simulink model "kamerol"  (R2021b)
settings: Solver=VariableStepAuto  StartTime=0.0  StopTime=10.0  RelTol=1e-3
undefined symbols (not defined in the file): admireDB
libraries: simulink_extras x104, simulink x24, sharedutil x1
(part 10 of 14)

== system kamerol/Aerodynamics/PitchMomentCoefficient/MachRegion2/Cpmdle/Subsystem ==
  angleOfAttack_deg : Inport
  dE : Inport  Port=2
  dN : Inport  Port=3
  tflow : Inport  Port=4
  tfhigh : Inport  Port=5
  lef_deg : Inport  Port=6
  " mach_nd_cnst" : Constant  Value=0.5
  CPMDLAL_ALFA : Lookup_n-D  NumberOfTableDimensions=1  BreakpointsForDimension1=admireDB.aerodata_sym.CPMDLAL.breakpoints.ALFA  BreakpointsForDimension3=[5, 7]  Table=admireDB.aerodata_sym.CPMDLAL.newTable  ExtrapMethod=Clip  InternalRulePriority=Speed  RndMeth=Simplest  InputSameDT=on
  CPMDLDEA_DE_ALFA : Lookup_n-D  BreakpointsForDimension1=admireDB.aerodata_sym.CPMDLDEA.breakpoints.ALFA  BreakpointsForDimension2=admireDB.aerodata_sym.CPMDLDEA.breakpoints.DE  BreakpointsForDimension3=[5, 7]  Table=admireDB.aerodata_sym.CPMDLDEA.newTable  ExtrapMethod=Clip  InternalRulePriority=Speed  RndMeth=Simplest  InputSameDT=on
      settings: InputPortMap=u0,u1
  CPMDLDNA_DN_ALFA : Lookup_n-D  BreakpointsForDimension1=admireDB.aerodata_sym.CPMDLDNA.breakpoints.ALFA  BreakpointsForDimension2=admireDB.aerodata_sym.CPMDLDNA.breakpoints.DN  BreakpointsForDimension3=[5, 7]  Table=admireDB.aerodata_sym.CPMDLDNA.newTable  ExtrapMethod=Clip  InternalRulePriority=Speed  RndMeth=Simplest  InputSameDT=on
      settings: InputPortMap=u0,u1
  CPMMDLEA_ALFA_DLE_M : Lookup_n-D  NumberOfTableDimensions=3  BreakpointsForDimension1=admireDB.aerodata_sym.CPMMDLEA.breakpoints.ALFA  BreakpointsForDimension2=admireDB.aerodata_sym.CPMMDLEA.breakpoints.DLE  BreakpointsForDimension3=admireDB.aerodata_sym.CPMMDLEA.breakpoints.M  Table=admireDB.aerodata_sym.CPMMDLEA.newTable  ExtrapMethod=Clip  InternalRulePriority=Speed  RndMeth=Simplest  InputSameDT=on
      settings: InputPortMap=u0,u1,u2
  Constant : Constant  Value=1/27
  Product : Product  Inputs=4
  Product1 : Product
  Sum : Sum  Inputs=+++
  Sum1 : Sum  Inputs=|++
  Out1 : Outport
  wires:
  Product1/1 -> Sum1/2
  Sum1/1 -> Out1/1
  tfhigh/1 -> Product1/1
  CPMMDLEA_ALFA_DLE_M/1 -> Product1/2
  angleOfAttack_deg/1 -> CPMDLAL_ALFA/1, CPMDLDEA_DE_ALFA/1, CPMDLDNA_DN_ALFA/1, CPMMDLEA_ALFA_DLE_M/1
  lef_deg/1 -> Product/3, CPMMDLEA_ALFA_DLE_M/2
  " mach_nd_cnst"/1 -> CPMMDLEA_ALFA_DLE_M/3
  tflow/1 -> Product/1
  dE/1 -> CPMDLDEA_DE_ALFA/2
  CPMDLDNA_DN_ALFA/1 -> Sum/3
  Sum/1 -> Product/2
  CPMDLAL_ALFA/1 -> Sum/1
  CPMDLDEA_DE_ALFA/1 -> Sum/2
  Product/1 -> Sum1/1
  dN/1 -> CPMDLDNA_DN_ALFA/2
  Constant/1 -> Product/4

== system kamerol/Aerodynamics/PitchMomentCoefficient/MachRegion2/Cpmdle/Subsystem1 ==
  qacorr : Inport
  mach_nd : Inport  Port=2
  CPMEDLEI_QA_M : Lookup_n-D  BreakpointsForDimension1=admireDB.aerodata_sym.CPMEDLEI.breakpoints.M  BreakpointsForDimension2=admireDB.aerodata_sym.CPMEDLEI.breakpoints.QA  BreakpointsForDimension3=[5, 7]  Table=admireDB.aerodata_sym.CPMEDLEI.newTable  ExtrapMethod=Clip  InternalRulePriority=Speed  RndMeth=Simplest  InputSameDT=on
      settings: InputPortMap=u0,u1
  CPMEDLEY_QA_M : Lookup_n-D  BreakpointsForDimension1=admireDB.aerodata_sym.CPMEDLEY.breakpoints.M  BreakpointsForDimension2=admireDB.aerodata_sym.CPMEDLEY.breakpoints.QA  BreakpointsForDimension3=[5, 7]  Table=admireDB.aerodata_sym.CPMEDLEY.newTable  ExtrapMethod=Clip  InternalRulePriority=Speed  RndMeth=Simplest  InputSameDT=on
      settings: InputPortMap=u0,u1
  Sum1 : Sum  Inputs=|++
  Out1 : Outport
  wires:
  mach_nd/1 -> CPMEDLEY_QA_M/1, CPMEDLEI_QA_M/1
  CPMEDLEY_QA_M/1 -> Sum1/2
  CPMEDLEI_QA_M/1 -> Sum1/1
  qacorr/1 -> CPMEDLEY_QA_M/2, CPMEDLEI_QA_M/2
  Sum1/1 -> Out1/1

== system kamerol/Aerodynamics/PitchMomentCoefficient/MachRegion2/Cpmdn/CPMDNAL_CPMMDNA ==
  dN : Inport
  angleOfAttack_deg : Inport  Port=2
  tflow : Inport  Port=3
  tfhigh : Inport  Port=4
  CPMDNAL_DN_ALFA : Lookup_n-D  BreakpointsForDimension1=admireDB.aerodata_sym.CPMDNAL.breakpoints.ALFA  BreakpointsForDimension2=admireDB.aerodata_sym.CPMDNAL.breakpoints.DN  BreakpointsForDimension3=[5, 7]  Table=admireDB.aerodata_sym.CPMDNAL.newTable  ExtrapMethod=Clip  InternalRulePriority=Speed  RndMeth=Simplest  InputSameDT=on
      settings: InputPortMap=u0,u1
  CPMMDNA_ALFA_DN_M : Lookup_n-D  NumberOfTableDimensions=3  BreakpointsForDimension1=admireDB.aerodata_sym.CPMMDNA.breakpoints.ALFA  BreakpointsForDimension2=admireDB.aerodata_sym.CPMMDNA.breakpoints.DN  BreakpointsForDimension3=admireDB.aerodata_sym.CPMMDNA.breakpoints.M  Table=admireDB.aerodata_sym.CPMMDNA.newTable  ExtrapMethod=Clip  InternalRulePriority=Speed  RndMeth=Simplest  InputSameDT=on
      settings: InputPortMap=u0,u1,u2
  Product : Product
  Product1 : Product
  Sum : Sum  Inputs=|++
  mach_nd_cnst : Constant  Value=0.5
  Out1 : Outport
  wires:
  Product1/1 -> Sum/2
  tfhigh/1 -> Product1/1
  Product/1 -> Sum/1
  tflow/1 -> Product/2
  mach_nd_cnst/1 -> CPMMDNA_ALFA_DN_M/3
  Sum/1 -> Out1/1
  angleOfAttack_deg/1 -> CPMDNAL_DN_ALFA/1, CPMMDNA_ALFA_DN_M/1
  CPMDNAL_DN_ALFA/1 -> Product/1
  dN/1 -> CPMDNAL_DN_ALFA/2, CPMMDNA_ALFA_DN_M/2
  CPMMDNA_ALFA_DN_M/1 -> Product1/2

== system kamerol/Aerodynamics/PitchMomentCoefficient/MachRegion2/Cpmq/Subsystem ==
  tflow : Inport
  angleOfAttack_deg : Inport  Port=2
  dN : Inport  Port=3
  tfhigh : Inport  Port=4
  CPMQAL_ALFA : Lookup_n-D  NumberOfTableDimensions=1  BreakpointsForDimension1=admireDB.aerodata_sym.CPMQAL.breakpoints.ALFA  BreakpointsForDimension3=[5, 7]  Table=admireDB.aerodata_sym.CPMQAL.newTable  ExtrapMethod=Clip  InternalRulePriority=Speed  RndMeth=Simplest  InputSameDT=on
  CPMQAM_ALFA_M : Lookup_n-D  BreakpointsForDimension1=admireDB.aerodata_sym.CPMQAM.breakpoints.M  BreakpointsForDimension2=admireDB.aerodata_sym.CPMQAM.breakpoints.ALFA  BreakpointsForDimension3=[5, 7]  Table=admireDB.aerodata_sym.CPMQAM.newTable  ExtrapMethod=Clip  InternalRulePriority=Speed  RndMeth=Simplest  InputSameDT=on
      settings: InputPortMap=u0,u1
  CPMQDNAL_DN_ALFA : Lookup_n-D  BreakpointsForDimension1=admireDB.aerodata_sym.CPMQDNAL.breakpoints.ALFA  BreakpointsForDimension2=admireDB.aerodata_sym.CPMQDNAL.breakpoints.DN  BreakpointsForDimension3=[5, 7]  Table=admireDB.aerodata_sym.CPMQDNAL.newTable  ExtrapMethod=Clip  InternalRulePriority=Speed  RndMeth=Simplest  InputSameDT=on
      settings: InputPortMap=u0,u1
  Product1 : Product
  Product2 : Product
  Sum : Sum  Inputs=++|
  Sum1 : Sum  Inputs=|++
  mach_nd_cnst : Constant  Value=0.5
  Out1 : Outport
  wires:
  dN/1 -> CPMQDNAL_DN_ALFA/2
  tfhigh/1 -> Product2/2
  Sum1/1 -> Out1/1
  tflow/1 -> Product1/1
  angleOfAttack_deg/1 -> CPMQAM_ALFA_M/2, CPMQDNAL_DN_ALFA/1, CPMQAL_ALFA/1
  Product2/1 -> Sum1/2
  CPMQAM_ALFA_M/1 -> Product2/1
  CPMQAL_ALFA/1 -> Sum/1
  mach_nd_cnst/1 -> CPMQAM_ALFA_M/1
  Sum/1 -> Product1/2
  Product1/1 -> Sum1/1
  CPMQDNAL_DN_ALFA/1 -> Sum/2

== system kamerol/Aerodynamics/PitchMomentCoefficient/MachRegion3/Cpmdei/Subsystem ==
  dEI : Inport
  angleOfAttack_deg : Inport  Port=2
  eieff : Inport  Port=3
  mach_nd : Inport  Port=4
  CPMMDEA_ALFA_DE_M : Lookup_n-D  NumberOfTableDimensions=3  BreakpointsForDimension1=admireDB.aerodata_sym.CPMMDEA.breakpoints.ALFA  BreakpointsForDimension2=admireDB.aerodata_sym.CPMMDEA.breakpoints.DE  BreakpointsForDimension3=admireDB.aerodata_sym.CPMMDEA.breakpoints.M  Table=admireDB.aerodata_sym.CPMMDEA.newTable  ExtrapMethod=Clip  InternalRulePriority=Speed  RndMeth=Simplest  InputSameDT=on
      settings: InputPortMap=u0,u1,u2
  CPMMDEA_ALFA_DE_M1 : Lookup_n-D  NumberOfTableDimensions=3  BreakpointsForDimension1=admireDB.aerodata_sym.CPMMDEA.breakpoints.ALFA  BreakpointsForDimension2=admireDB.aerodata_sym.CPMMDEA.breakpoints.DE  BreakpointsForDimension3=admireDB.aerodata_sym.CPMMDEA.breakpoints.M  Table=admireDB.aerodata_sym.CPMMDEA.newTable  ExtrapMethod=Clip  InternalRulePriority=Speed  RndMeth=Simplest  InputSameDT=on
      settings: InputPortMap=u0,u1,u2
  Constant : Constant  Value=0
  Product : Product
  Sum : Sum  Inputs=|+-
  Out1 : Outport
  wires:
  Constant/1 -> CPMMDEA_ALFA_DE_M1/2
  mach_nd/1 -> CPMMDEA_ALFA_DE_M1/3, CPMMDEA_ALFA_DE_M/3
  eieff/1 -> Product/2
  angleOfAttack_deg/1 -> CPMMDEA_ALFA_DE_M/1, CPMMDEA_ALFA_DE_M1/1
  Sum/1 -> Product/1
  CPMMDEA_ALFA_DE_M1/1 -> Sum/2
  CPMMDEA_ALFA_DE_M/1 -> Sum/1
  Product/1 -> Out1/1
  dEI/1 -> CPMMDEA_ALFA_DE_M/2

== system kamerol/Aerodynamics/PitchMomentCoefficient/MachRegion3/Cpmdey/Subsystem ==
  dEY : Inport
  angleOfAttack_deg : Inport  Port=2
  eoeff : Inport  Port=3
  mach_nd : Inport  Port=4
  CPMMDEA_ALFA_DE_M : Lookup_n-D  NumberOfTableDimensions=3  BreakpointsForDimension1=admireDB.aerodata_sym.CPMMDEA.breakpoints.ALFA  BreakpointsForDimension2=admireDB.aerodata_sym.CPMMDEA.breakpoints.DE  BreakpointsForDimension3=admireDB.aerodata_sym.CPMMDEA.breakpoints.M  Table=admireDB.aerodata_sym.CPMMDEA.newTable  ExtrapMethod=Clip  InternalRulePriority=Speed  RndMeth=Simplest  InputSameDT=on
      settings: InputPortMap=u0,u1,u2
  CPMMDEA_ALFA_DE_M1 : Lookup_n-D  NumberOfTableDimensions=3  BreakpointsForDimension1=admireDB.aerodata_sym.CPMMDEA.breakpoints.ALFA  BreakpointsForDimension2=admireDB.aerodata_sym.CPMMDEA.breakpoints.DE  BreakpointsForDimension3=admireDB.aerodata_sym.CPMMDEA.breakpoints.M  Table=admireDB.aerodata_sym.CPMMDEA.newTable  ExtrapMethod=Clip  InternalRulePriority=Speed  RndMeth=Simplest  InputSameDT=on
      settings: InputPortMap=u0,u1,u2
  Constant : Constant  Value=0
  Product : Product
  Sum : Sum  Inputs=|+-
  Out1 : Outport
  wires:
  dEY/1 -> CPMMDEA_ALFA_DE_M/2
  Product/1 -> Out1/1
  CPMMDEA_ALFA_DE_M/1 -> Sum/1
  CPMMDEA_ALFA_DE_M1/1 -> Sum/2
  Sum/1 -> Product/1
  angleOfAttack_deg/1 -> CPMMDEA_ALFA_DE_M1/1, CPMMDEA_ALFA_DE_M/1
  eoeff/1 -> Product/2
  mach_nd/1 -> CPMMDEA_ALFA_DE_M/3, CPMMDEA_ALFA_DE_M1/3
  Constant/1 -> CPMMDEA_ALFA_DE_M1/2

== system kamerol/Aerodynamics/PitchMomentCoefficient/MachRegion3/Cpmdle/Subsystem1 ==
  <qacorr> : Inport
  <mach_nd> : Inport  Port=2
  CPMEDLEI_QA_M : Lookup_n-D  BreakpointsForDimension1=admireDB.aerodata_sym.CPMEDLEI.breakpoints.M  BreakpointsForDimension2=admireDB.aerodata_sym.CPMEDLEI.breakpoints.QA  BreakpointsForDimension3=[5, 7]  Table=admireDB.aerodata_sym.CPMEDLEI.newTable  ExtrapMethod=Clip  InternalRulePriority=Speed  RndMeth=Simplest  InputSameDT=on
      settings: InputPortMap=u0,u1
  CPMEDLEY_QA_M : Lookup_n-D  BreakpointsForDimension1=admireDB.aerodata_sym.CPMEDLEY.breakpoints.M  BreakpointsForDimension2=admireDB.aerodata_sym.CPMEDLEY.breakpoints.QA  BreakpointsForDimension3=[5, 7]  Table=admireDB.aerodata_sym.CPMEDLEY.newTable  ExtrapMethod=Clip  InternalRulePriority=Speed  RndMeth=Simplest  InputSameDT=on
      settings: InputPortMap=u0,u1
  Sum1 : Sum  Inputs=|++
  Out1 : Outport
  wires:
  <mach_nd>/1 -> CPMEDLEY_QA_M/1, CPMEDLEI_QA_M/1
  CPMEDLEY_QA_M/1 -> Sum1/2
  CPMEDLEI_QA_M/1 -> Sum1/1
  <qacorr>/1 -> CPMEDLEY_QA_M/2, CPMEDLEI_QA_M/2
  Sum1/1 -> Out1/1

== system kamerol/Aerodynamics/RollMomentCoefficient/MachRegion1/Crmbasic/Crmbasic_ ==
  angleOfAttack_deg : Inport
  Abs : Abs
  CRMZERO_ALFA : Lookup_n-D  NumberOfTableDimensions=1  BreakpointsForDimension1=admireDB.aerodata_asym_ext.CRMZERO.breakpoints.ALFA  BreakpointsForDimension3=[5, 7]  Table=admireDB.aerodata_asym_ext.CRMZERO.newTable  ExtrapMethod=Clip  InternalRulePriority=Speed  RndMeth=Simplest  InputSameDT=on
  Crmbasic : Outport
  wires:
  Abs/1 -> CRMZERO_ALFA/1
  angleOfAttack_deg/1 -> Abs/1
  CRMZERO_ALFA/1 -> Crmbasic/1

== system kamerol/Aerodynamics/RollMomentCoefficient/MachRegion1/Crmbde/Crmbde_ ==
  angleOfAttack_deg : Inport
  dN : Inport  Port=2
  dEI : Inport  Port=3
  angleOfSideslip_deg : Inport  Port=4
  dEY : Inport  Port=5
  eieff : Inport  Port=6
  eoeff : Inport  Port=7
  Abs : Abs
  CRMDEB_ALFA_DN_DE_BETA : Lookup_n-D  NumberOfTableDimensions=4  BreakpointsForDimension1=admireDB.aerodata_asym_ext.CRMDEB.breakpoints.ALFA  BreakpointsForDimension2=admireDB.aerodata_asym_ext.CRMDEB.breakpoints.DN  BreakpointsForDimension3=admireDB.aerodata_asym_ext.CRMDEB.breakpoints.DE  BreakpointsForDimension4=admireDB.aerodata_asym_ext.CRMDEB.breakpoints.BETA  Table=admireDB.aerodata_asym_ext.CRMDEB.newTable  ExtrapMethod=Clip  InternalRulePriority=Speed  RndMeth=Simplest  InputSameDT=on
      settings: InputPortMap=u0,u1,u2,u3
  CRMDEB_ALFA_DN_DE_BETA_1 : Lookup_n-D  NumberOfTableDimensions=4  BreakpointsForDimension1=admireDB.aerodata_asym_ext.CRMDEB.breakpoints.ALFA  BreakpointsForDimension2=admireDB.aerodata_asym_ext.CRMDEB.breakpoints.DN  BreakpointsForDimension3=admireDB.aerodata_asym_ext.CRMDEB.breakpoints.DE  BreakpointsForDimension4=admireDB.aerodata_asym_ext.CRMDEB.breakpoints.BETA  Table=admireDB.aerodata_asym_ext.CRMDEB.newTable  ExtrapMethod=Clip  InternalRulePriority=Speed  RndMeth=Simplest  InputSameDT=on
      settings: InputPortMap=u0,u1,u2,u3
  Product : Product  Inputs=**
  Product1 : Product  Inputs=**
  Product2 : Product
  Sign : Signum
  Sum : Sum  Inputs=|++
  Crmbde : Outport
  wires:
  dEY/1 -> CRMDEB_ALFA_DN_DE_BETA_1/3
  dEI/1 -> CRMDEB_ALFA_DN_DE_BETA/3
  dN/1 -> CRMDEB_ALFA_DN_DE_BETA_1/2, CRMDEB_ALFA_DN_DE_BETA/2
  angleOfAttack_deg/1 -> CRMDEB_ALFA_DN_DE_BETA_1/1, CRMDEB_ALFA_DN_DE_BETA/1
  Sign/1 -> Product2/1
  Product2/1 -> Crmbde/1
  Product1/1 -> Sum/2
  Product/1 -> Sum/1
  Sum/1 -> Product2/2
  eoeff/1 -> Product1/1
  eieff/1 -> Product/2
  CRMDEB_ALFA_DN_DE_BETA_1/1 -> Product1/2
  CRMDEB_ALFA_DN_DE_BETA/1 -> Product/1
  Abs/1 -> CRMDEB_ALFA_DN_DE_BETA_1/4, CRMDEB_ALFA_DN_DE_BETA/4
  angleOfSideslip_deg/1 -> Abs/1, Sign/1

== system kamerol/Aerodynamics/RollMomentCoefficient/MachRegion1/Crmbdle/Crmbdle_ ==
  dLE : Inport
  angleOfSideslip_deg : Inport  Port=2
  dEI : Inport  Port=3
  angleOfAttack_deg : Inport  Port=4
  dEY : Inport  Port=5
  eieff : Inport  Port=6
  eoeff : Inport  Port=7
  Abs : Abs
  CRMDLEB_ALFA_DE_BETA_DLE : Lookup_n-D  NumberOfTableDimensions=4  BreakpointsForDimension1=admireDB.aerodata_asym_ext.CRMDLEB.breakpoints.ALFA  BreakpointsForDimension2=admireDB.aerodata_asym_ext.CRMDLEB.breakpoints.DE  BreakpointsForDimension3=admireDB.aerodata_asym_ext.CRMDLEB.breakpoints.BETA  BreakpointsForDimension4=admireDB.aerodata_asym_ext.CRMDLEB.breakpoints.DLE  Table=admireDB.aerodata_asym_ext.CRMDLEB.newTable  ExtrapMethod=Clip  InternalRulePriority=Speed  RndMeth=Simplest  InputSameDT=on
      settings: InputPortMap=u0,u1,u2,u3
  CRMDLEB_ALFA_DE_BETA_DLE_1 : Lookup_n-D  NumberOfTableDimensions=4  BreakpointsForDimension1=admireDB.aerodata_asym_ext.CRMDLEB.breakpoints.ALFA  BreakpointsForDimension2=admireDB.aerodata_asym_ext.CRMDLEB.breakpoints.DE  BreakpointsForDimension3=admireDB.aerodata_asym_ext.CRMDLEB.breakpoints.BETA  BreakpointsForDimension4=admireDB.aerodata_asym_ext.CRMDLEB.breakpoints.DLE  Table=admireDB.aerodata_asym_ext.CRMDLEB.newTable  ExtrapMethod=Clip  InternalRulePriority=Speed  RndMeth=Simplest  InputSameDT=on
      settings: InputPortMap=u0,u1,u2,u3
  Product1 : Product  Inputs=**
  Product2 : Product  Inputs=**
  Product3 : Product
  Sign : Signum
  Sum : Sum  Inputs=|++
  Crmbdle : Outport
  wires:
  dEY/1 -> CRMDLEB_ALFA_DE_BETA_DLE_1/2
  dEI/1 -> CRMDLEB_ALFA_DE_BETA_DLE/2
  Abs/1 -> CRMDLEB_ALFA_DE_BETA_DLE_1/3, CRMDLEB_ALFA_DE_BETA_DLE/3
  dLE/1 -> CRMDLEB_ALFA_DE_BETA_DLE_1/4, CRMDLEB_ALFA_DE_BETA_DLE/4
  CRMDLEB_ALFA_DE_BETA_DLE/1 -> Product1/1
  eoeff/1 -> Product2/1
  Product1/1 -> Sum/1
  Sum/1 -> Product3/2
  CRMDLEB_ALFA_DE_BETA_DLE_1/1 -> Product2/2
  Sign/1 -> Product3/1
  eieff/1 -> Product1/2
  Product2/1 -> Sum/2
  angleOfSideslip_deg/1 -> Abs/1, Sign/1
  angleOfAttack_deg/1 -> CRMDLEB_ALFA_DE_BETA_DLE_1/1, CRMDLEB_ALFA_DE_BETA_DLE/1
  Product3/1 -> Crmbdle/1

== system kamerol/Aerodynamics/RollMomentCoefficient/MachRegion1/Crmbdn/Crmbdn_ ==
  angleOfAttack_deg : Inport
  dN : Inport  Port=2
  angleOfSideslip_deg : Inport  Port=3
  Abs : Abs
  CRMDNB_ALFA_DN_BETA : Lookup_n-D  NumberOfTableDimensions=3  BreakpointsForDimension1=admireDB.aerodata_asym_ext.CRMDNB.breakpoints.ALFA  BreakpointsForDimension2=admireDB.aerodata_asym_ext.CRMDNB.breakpoints.DN  BreakpointsForDimension3=admireDB.aerodata_asym_ext.CRMDNB.breakpoints.BETA  Table=admireDB.aerodata_asym_ext.CRMDNB.newTable  ExtrapMethod=Clip  InternalRulePriority=Speed  RndMeth=Simplest  InputSameDT=on
      settings: InputPortMap=u0,u1,u2
  Product : Product
  Sign : Signum
  Crmbdn : Outport
  wires:
  Sign/1 -> Product/2
  CRMDNB_ALFA_DN_BETA/1 -> Product/1
  angleOfSideslip_deg/1 -> Abs/1, Sign/1
  angleOfAttack_deg/1 -> CRMDNB_ALFA_DN_BETA/1
  dN/1 -> CRMDNB_ALFA_DN_BETA/2
  Abs/1 -> CRMDNB_ALFA_DN_BETA/3
  Product/1 -> Crmbdn/1

== system kamerol/Aerodynamics/RollMomentCoefficient/MachRegion1/Crmbeta/Crmbeta_ ==
  angleOfSideslip_deg : Inport
  angleOfAttack_deg : Inport  Port=2
  qacorr : Inport  Port=3
  mach_nd : Inport  Port=4
  Abs : Abs
  CRMBAL_BETA_ALFA : Lookup_n-D  BreakpointsForDimension1=admireDB.aerodata_asym_ext.CRMBAL.breakpoints.ALFA  BreakpointsForDimension2=admireDB.aerodata_asym_ext.CRMBAL.breakpoints.BETA  BreakpointsForDimension3=[5, 7]  Table=admireDB.aerodata_asym_ext.CRMBAL.newTable  ExtrapMethod=Clip  InternalRulePriority=Speed  RndMeth=Simplest  InputSameDT=on
      settings: InputPortMap=u0,u1
  CRMEB_QA_M : Lookup_n-D  BreakpointsForDimension1=admireDB.aerodata_asym_ext.CRMEB.breakpoints.M  BreakpointsForDimension2=admireDB.aerodata_asym_ext.CRMEB.breakpoints.QA  BreakpointsForDimension3=[5, 7]  Table=admireDB.aerodata_asym_ext.CRMEB.newTable  ExtrapMethod=Clip  InternalRulePriority=Speed  RndMeth=Simplest  InputSameDT=on
      settings: InputPortMap=u0,u1
  Degrees to Radians : simulink_extras/Transformations/Degrees to Radians
  Product : Product
  Product1 : Product
  Sign : Signum
  Sum : Sum  Inputs=|++
  Crmbeta : Outport
  wires:
  Sum/1 -> Crmbeta/1
  Product1/1 -> Sum/2
  Degrees to Radians/1 -> Product1/1
  CRMEB_QA_M/1 -> Product1/2
  Product/1 -> Sum/1
  Abs/1 -> CRMBAL_BETA_ALFA/2
  Sign/1 -> Product/1
  CRMBAL_BETA_ALFA/1 -> Product/2
  angleOfSideslip_deg/1 -> Abs/1, Sign/1, Degrees to Radians/1
  mach_nd/1 -> CRMEB_QA_M/1
  angleOfAttack_deg/1 -> CRMBAL_BETA_ALFA/1
  qacorr/1 -> CRMEB_QA_M/2

== system kamerol/Aerodynamics/RollMomentCoefficient/MachRegion1/Crmbetad/Crmbetad_ ==
  angleOfAttack_deg : Inport
  betad : Inport  Port=2
  CRMBDL_ALFA : Lookup_n-D  NumberOfTableDimensions=1  BreakpointsForDimension1=admireDB.aerodata_asym_ext.CRMBDL.breakpoints.ALFA  BreakpointsForDimension3=[5, 7]  Table=admireDB.aerodata_asym_ext.CRMBDL.newTable  ExtrapMethod=Clip  InternalRulePriority=Speed  RndMeth=Simplest  InputSameDT=on
  Product : Product  Inputs=**
  Crmbetad : Outport
  wires:
  angleOfAttack_deg/1 -> CRMBDL_ALFA/1
  Product/1 -> Crmbetad/1
  CRMBDL_ALFA/1 -> Product/1
  betad/1 -> Product/2

== system kamerol/Aerodynamics/RollMomentCoefficient/MachRegion1/Crmblg/Crmblg_ ==
  dLG : Inport
  angleOfAttack_deg : Inport  Port=2
  angleOfSideslip_deg : Inport  Port=3
  CRMBLST_NG_DOOR_ALFA : Lookup_n-D  BreakpointsForDimension1=admireDB.aerodata_asym_ext.CRMBLST.breakpoints.ALFA  BreakpointsForDimension2=admireDB.aerodata_asym_ext.CRMBLST.breakpoints.NG_DOOR  BreakpointsForDimension3=[5, 7]  Table=admireDB.aerodata_asym_ext.CRMBLST.newTable  ExtrapMethod=Clip  InternalRulePriority=Speed  RndMeth=Simplest  InputSameDT=on
      settings: InputPortMap=u0,u1
  Degrees to Radians : simulink_extras/Transformations/Degrees to Radians
  Product : Product  Inputs=3
  Crmblg : Outport
  wires:
  Degrees to Radians/1 -> Product/3
  CRMBLST_NG_DOOR_ALFA/1 -> Product/2
  dLG/1 -> CRMBLST_NG_DOOR_ALFA/2, Product/1
  angleOfAttack_deg/1 -> CRMBLST_NG_DOOR_ALFA/1
  Product/1 -> Crmblg/1
  angleOfSideslip_deg/1 -> Degrees to Radians/1

== system kamerol/Aerodynamics/RollMomentCoefficient/MachRegion1/Crmdai/Crmdai_ ==
  dAI : Inport
  angleOfAttack_deg : Inport  Port=2
  dEI : Inport  Port=3
  eieff : Inport  Port=4
  qacorr : Inport  Port=5
  mach_nd : Inport  Port=6
  Abs : Abs
  CRMDAAL_DA_ALFA : Lookup_n-D  BreakpointsForDimension1=admireDB.aerodata_asym_ext.CRMDAAL.breakpoints.ALFA  BreakpointsForDimension2=admireDB.aerodata_asym_ext.CRMDAAL.breakpoints.DA  BreakpointsForDimension3=[5, 7]  Table=admireDB.aerodata_asym_ext.CRMDAAL.newTable  ExtrapMethod=Clip  InternalRulePriority=Speed  RndMeth=Simplest  InputSameDT=on
      settings: InputPortMap=u0,u1
  CRMDAL_DE_ALFA : Lookup_n-D  BreakpointsForDimension1=admireDB.aerodata_asym_ext.CRMDAL.breakpoints.ALFA  BreakpointsForDimension2=admireDB.aerodata_asym_ext.CRMDAL.breakpoints.DE  BreakpointsForDimension3=[5, 7]  Table=admireDB.aerodata_asym_ext.CRMDAL.newTable  ExtrapMethod=Clip  InternalRulePriority=Speed  RndMeth=Simplest  InputSameDT=on
      settings: InputPortMap=u0,u1
  CRMDAL_DE_ALFA_1 : Lookup_n-D  BreakpointsForDimension1=admireDB.aerodata_asym_ext.CRMDAL.breakpoints.ALFA  BreakpointsForDimension2=admireDB.aerodata_asym_ext.CRMDAL.breakpoints.DE  BreakpointsForDimension3=[5, 7]  Table=admireDB.aerodata_asym_ext.CRMDAL.newTable  ExtrapMethod=Clip  InternalRulePriority=Speed  RndMeth=Simplest  InputSameDT=on
      settings: InputPortMap=u0,u1
  CRMEDAI_QA_M : Lookup_n-D  BreakpointsForDimension1=admireDB.aerodata_asym_ext.CRMEDAI.breakpoints.M  BreakpointsForDimension2=admireDB.aerodata_asym_ext.CRMEDAI.breakpoints.QA  BreakpointsForDimension3=[5, 7]  Table=admireDB.aerodata_asym_ext.CRMEDAI.newTable  ExtrapMethod=Clip  InternalRulePriority=Speed  RndMeth=Simplest  InputSameDT=on
      settings: InputPortMap=u0,u1
  Degrees to Radians : simulink_extras/Transformations/Degrees to Radians
  Product : Product
  Product1 : Product
  Product2 : Product  Inputs=3
  Sign : Signum
  Sum : Sum  Inputs=|+-
  Sum1 : Sum  Inputs=|++
  dE_cnst : Constant  Value=0.0
  Crmdai : Outport
  wires:
  CRMEDAI_QA_M/1 -> Product2/3
  qacorr/1 -> CRMEDAI_QA_M/2
  mach_nd/1 -> CRMEDAI_QA_M/1
  eieff/1 -> Product2/2
  Sum1/1 -> Product2/1
  Product/1 -> Sum1/2
  Product1/1 -> Sum1/1
  Sign/1 -> Product1/1
  CRMDAAL_DA_ALFA/1 -> Product1/2
  Degrees to Radians/1 -> Product/1
  Sum/1 -> Product/2
  CRMDAL_DE_ALFA_1/1 -> Sum/2
  CRMDAL_DE_ALFA/1 -> Sum/1
  dEI/1 -> CRMDAL_DE_ALFA/2
  dE_cnst/1 -> CRMDAL_DE_ALFA_1/2
  dAI/1 -> Abs/1, Sign/1, Degrees to Radians/1
  Abs/1 -> CRMDAAL_DA_ALFA/2
  angleOfAttack_deg/1 -> CRMDAAL_DA_ALFA/1, CRMDAL_DE_ALFA_1/1, CRMDAL_DE_ALFA/1
  Product2/1 -> Crmdai/1

== system kamerol/Aerodynamics/RollMomentCoefficient/MachRegion1/Crmdaib/Crmdaib_ ==
  angleOfAttack_deg : Inport
  dAI : Inport  Port=2
  angleOfSideslip_deg : Inport  Port=3
  eieff : Inport  Port=4
  Abs : Abs
  Abs1 : Abs
  Abs2 : Abs
  CRMDABAL_ALFA : Lookup_n-D  NumberOfTableDimensions=1  BreakpointsForDimension1=admireDB.aerodata_asym_ext.CRMDABAL.breakpoints.ALFA  BreakpointsForDimension3=[5, 7]  Table=admireDB.aerodata_asym_ext.CRMDABAL.newTable  ExtrapMethod=Clip  InternalRulePriority=Speed  RndMeth=Simplest  InputSameDT=on
  Constant : Constant  Value=30
  Constant1 : Constant  Value=20
  Product : Product  Inputs=**/*/*
  Crmdaib : Outport
  wires:
  eieff/1 -> Product/6
  Abs2/1 -> Product/4
  Constant1/1 -> Product/5
  angleOfSideslip_deg/1 -> Abs2/1
  Constant/1 -> Product/3
  Abs1/1 -> Product/2
  Abs/1 -> CRMDABAL_ALFA/1
  dAI/1 -> Abs1/1
  CRMDABAL_ALFA/1 -> Product/1
  angleOfAttack_deg/1 -> Abs/1
  Product/1 -> Crmdaib/1

== system kamerol/Aerodynamics/RollMomentCoefficient/MachRegion1/Crmday/Crmday_ ==
  dAY : Inport
  angleOfAttack_deg : Inport  Port=2
  dEY : Inport  Port=3
  eoeff : Inport  Port=4
  qacorr : Inport  Port=5
  mach_nd : Inport  Port=6
  Abs : Abs
  CRMDAAL_DA_ALFA : Lookup_n-D  BreakpointsForDimension1=admireDB.aerodata_asym_ext.CRMDAAL.breakpoints.ALFA  BreakpointsForDimension2=admireDB.aerodata_asym_ext.CRMDAAL.breakpoints.DA  BreakpointsForDimension3=[5, 7]  Table=admireDB.aerodata_asym_ext.CRMDAAL.newTable  ExtrapMethod=Clip  InternalRulePriority=Speed  RndMeth=Simplest  InputSameDT=on
      settings: InputPortMap=u0,u1
  CRMDAL_DE_ALFA : Lookup_n-D  BreakpointsForDimension1=admireDB.aerodata_asym_ext.CRMDAL.breakpoints.ALFA  BreakpointsForDimension2=admireDB.aerodata_asym_ext.CRMDAL.breakpoints.DE  BreakpointsForDimension3=[5, 7]  Table=admireDB.aerodata_asym_ext.CRMDAL.newTable  ExtrapMethod=Clip  InternalRulePriority=Speed  RndMeth=Simplest  InputSameDT=on
      settings: InputPortMap=u0,u1
  CRMDAL_DE_ALFA_1 : Lookup_n-D  BreakpointsForDimension1=admireDB.aerodata_asym_ext.CRMDAL.breakpoints.ALFA  BreakpointsForDimension2=admireDB.aerodata_asym_ext.CRMDAL.breakpoints.DE  BreakpointsForDimension3=[5, 7]  Table=admireDB.aerodata_asym_ext.CRMDAL.newTable  ExtrapMethod=Clip  InternalRulePriority=Speed  RndMeth=Simplest  InputSameDT=on
      settings: InputPortMap=u0,u1
  CRMEDAY_QA_M : Lookup_n-D  BreakpointsForDimension1=admireDB.aerodata_asym_ext.CRMEDAY.breakpoints.M  BreakpointsForDimension2=admireDB.aerodata_asym_ext.CRMEDAY.breakpoints.QA  BreakpointsForDimension3=[5, 7]  Table=admireDB.aerodata_asym_ext.CRMEDAY.newTable  ExtrapMethod=Clip  InternalRulePriority=Speed  RndMeth=Simplest  InputSameDT=on
      settings: InputPortMap=u0,u1
  Degrees to Radians : simulink_extras/Transformations/Degrees to Radians
  Product : Product
  Product1 : Product
  Product2 : Product  Inputs=3
  Sign : Signum
  Sum : Sum  Inputs=|+-
  Sum1 : Sum  Inputs=|++
  dE_cnst : Constant  Value=0.0
  Crmdai : Outport
  wires:
  dE_cnst/1 -> CRMDAL_DE_ALFA_1/2
  Product2/1 -> Crmdai/1
  angleOfAttack_deg/1 -> CRMDAL_DE_ALFA_1/1, CRMDAL_DE_ALFA/1, CRMDAAL_DA_ALFA/1
  Abs/1 -> CRMDAAL_DA_ALFA/2
  dAY/1 -> Abs/1, Sign/1, Degrees to Radians/1
  dEY/1 -> CRMDAL_DE_ALFA/2
  CRMDAL_DE_ALFA/1 -> Sum/1
  CRMDAL_DE_ALFA_1/1 -> Sum/2
  Sum/1 -> Product/2
  Degrees to Radians/1 -> Product/1
  CRMDAAL_DA_ALFA/1 -> Product1/2
  Sign/1 -> Product1/1
  Product1/1 -> Sum1/1
  Product/1 -> Sum1/2
  Sum1/1 -> Product2/1
  eoeff/1 -> Product2/2
  qacorr/1 -> CRMEDAY_QA_M/2
  mach_nd/1 -> CRMEDAY_QA_M/1
  CRMEDAY_QA_M/1 -> Product2/3

== system kamerol/Aerodynamics/RollMomentCoefficient/MachRegion1/Crmdayb/Crmdaib_ ==
  angleOfAttack_deg : Inport
  dAY : Inport  Port=2
  angleOfSideslip_deg : Inport  Port=3
  eoeff : Inport  Port=4
  Abs : Abs
  Abs1 : Abs
  Abs2 : Abs
  CRMDABAL_ALFA : Lookup_n-D  NumberOfTableDimensions=1  BreakpointsForDimension1=admireDB.aerodata_asym_ext.CRMDABAL.breakpoints.ALFA  BreakpointsForDimension3=[5, 7]  Table=admireDB.aerodata_asym_ext.CRMDABAL.newTable  ExtrapMethod=Clip  InternalRulePriority=Speed  RndMeth=Simplest  InputSameDT=on
  Constant : Constant  Value=30
  Constant1 : Constant  Value=20
  Product : Product  Inputs=**/*/*
  Crmdaib : Outport
  wires:
  Product/1 -> Crmdaib/1
  angleOfAttack_deg/1 -> Abs/1
  CRMDABAL_ALFA/1 -> Product/1
  dAY/1 -> Abs1/1
  Abs/1 -> CRMDABAL_ALFA/1
  Abs1/1 -> Product/2
  Constant/1 -> Product/3
  angleOfSideslip_deg/1 -> Abs2/1
  Constant1/1 -> Product/5
  Abs2/1 -> Product/4
  eoeff/1 -> Product/6

== system kamerol/Aerodynamics/RollMomentCoefficient/MachRegion1/Crmdna/Crmdna_ ==
  dNE : Inport
  angleOfAttack_deg : Inport  Port=2
  dNA : Inport  Port=3
  CRMDNAAL_DNE_ALFA : Lookup_n-D  BreakpointsForDimension1=admireDB.aerodata_asym_ext.CRMDNAAL.breakpoints.ALFA  BreakpointsForDimension2=admireDB.aerodata_asym_ext.CRMDNAAL.breakpoints.DNE  BreakpointsForDimension3=[5, 7]  Table=admireDB.aerodata_asym_ext.CRMDNAAL.newTable  ExtrapMethod=Clip  InternalRulePriority=Speed  RndMeth=Simplest  InputSameDT=on
      settings: InputPortMap=u0,u1
  Degrees to Radians : simulink_extras/Transformations/Degrees to Radians
  Product : Product  Inputs=**
  Crmdna : Outport
  wires:
  Degrees to Radians/1 -> Product/2
  CRMDNAAL_DNE_ALFA/1 -> Product/1
  dNA/1 -> Degrees to Radians/1
  angleOfAttack_deg/1 -> CRMDNAAL_DNE_ALFA/1
  dNE/1 -> CRMDNAAL_DNE_ALFA/2
  Product/1 -> Crmdna/1

== system kamerol/Aerodynamics/RollMomentCoefficient/MachRegion1/Crmdr/Crmdr_ ==
  angleOfAttack_deg : Inport
  dR : Inport  Port=2
  angleOfSideslip_deg : Inport  Port=3
  qacorr : Inport  Port=4
  mach_nd : Inport  Port=5
  Abs : Abs
  CRMBDRAL_ALFA_DR_BETA : Lookup_n-D  NumberOfTableDimensions=3  BreakpointsForDimension1=admireDB.aerodata_asym_ext.CRMBDRAL.breakpoints.ALFA  BreakpointsForDimension2=admireDB.aerodata_asym_ext.CRMBDRAL.breakpoints.DR  BreakpointsForDimension3=admireDB.aerodata_asym_ext.CRMBDRAL.breakpoints.BETA  Table=admireDB.aerodata_asym_ext.CRMBDRAL.newTable  ExtrapMethod=Clip  InternalRulePriority=Speed  RndMeth=Simplest  InputSameDT=on
      settings: InputPortMap=u0,u1,u2
  CRMEDR_QA_M : Lookup_n-D  BreakpointsForDimension1=admireDB.aerodata_asym_ext.CRMEDR.breakpoints.M  BreakpointsForDimension2=admireDB.aerodata_asym_ext.CRMEDR.breakpoints.QA  BreakpointsForDimension3=[5, 7]  Table=admireDB.aerodata_asym_ext.CRMEDR.newTable  ExtrapMethod=Clip  InternalRulePriority=Speed  RndMeth=Simplest  InputSameDT=on
      settings: InputPortMap=u0,u1
  Product : Product
  Crmdr : Outport
  wires:
  CRMBDRAL_ALFA_DR_BETA/1 -> Product/1
  CRMEDR_QA_M/1 -> Product/2
  angleOfAttack_deg/1 -> CRMBDRAL_ALFA_DR_BETA/1
  angleOfSideslip_deg/1 -> Abs/1
  dR/1 -> CRMBDRAL_ALFA_DR_BETA/2
  Abs/1 -> CRMBDRAL_ALFA_DR_BETA/3
  qacorr/1 -> CRMEDR_QA_M/2
  mach_nd/1 -> CRMEDR_QA_M/1
  Product/1 -> Crmdr/1

== system kamerol/Aerodynamics/RollMomentCoefficient/MachRegion1/Crmp/Crmp_ ==
  dN : Inport
  angleOfAttack_deg : Inport  Port=2
  qacorr : Inport  Port=3
  mach_nd : Inport  Port=4
  pc : Inport  Port=5
  CRMEP_QA_M : Lookup_n-D  BreakpointsForDimension1=admireDB.aerodata_asym_ext.CRMEP.breakpoints.M  BreakpointsForDimension2=admireDB.aerodata_asym_ext.CRMEP.breakpoints.QA  BreakpointsForDimension3=[5, 7]  Table=admireDB.aerodata_asym_ext.CRMEP.newTable  ExtrapMethod=Clip  InternalRulePriority=Speed  RndMeth=Simplest  InputSameDT=on
      settings: InputPortMap=u0,u1
  CRMPAL_DN_ALFA : Lookup_n-D  BreakpointsForDimension1=admireDB.aerodata_asym_ext.CRMPAL.breakpoints.ALFA  BreakpointsForDimension2=admireDB.aerodata_asym_ext.CRMPAL.breakpoints.DN  BreakpointsForDimension3=[5, 7]  Table=admireDB.aerodata_asym_ext.CRMPAL.newTable  ExtrapMethod=Clip  InternalRulePriority=Speed  RndMeth=Simplest  InputSameDT=on
      settings: InputPortMap=u0,u1
  Product : Product  Inputs=3
  Crmp : Outport
  wires:
  Product/1 -> Crmp/1
  pc/1 -> Product/2
  CRMEP_QA_M/1 -> Product/3
  CRMPAL_DN_ALFA/1 -> Product/1
  angleOfAttack_deg/1 -> CRMPAL_DN_ALFA/1
  dN/1 -> CRMPAL_DN_ALFA/2
  mach_nd/1 -> CRMEP_QA_M/1
  qacorr/1 -> CRMEP_QA_M/2

== system kamerol/Aerodynamics/RollMomentCoefficient/MachRegion1/Crmpbeta/Crmpbeta_ ==
  angleOfSideslip_deg : Inport
  angleOfAttack_deg : Inport  Port=2
  pc : Inport  Port=3
  Abs : Abs
  CRMPBA_BETA_ALFA : Lookup_n-D  BreakpointsForDimension1=admireDB.aerodata_asym_ext.CRMPBA.breakpoints.ALFA  BreakpointsForDimension2=admireDB.aerodata_asym_ext.CRMPBA.breakpoints.BETA  BreakpointsForDimension3=[5, 7]  Table=admireDB.aerodata_asym_ext.CRMPBA.newTable  ExtrapMethod=Clip  InternalRulePriority=Speed  RndMeth=Simplest  InputSameDT=on
      settings: InputPortMap=u0,u1
  Product : Product  Inputs=**
  Crmpbeta : Outport
  wires:
  Abs/1 -> CRMPBA_BETA_ALFA/2
  CRMPBA_BETA_ALFA/1 -> Product/1
  angleOfSideslip_deg/1 -> Abs/1
  angleOfAttack_deg/1 -> CRMPBA_BETA_ALFA/1
  pc/1 -> Product/2
  Product/1 -> Crmpbeta/1

== system kamerol/Aerodynamics/RollMomentCoefficient/MachRegion1/Crmr/Crmr_ ==
  dN : Inport
  angleOfAttack_deg : Inport  Port=2
  rc : Inport  Port=3
  CRMRAL_DN_ALFA : Lookup_n-D  BreakpointsForDimension1=admireDB.aerodata_asym_ext.CRMRAL.breakpoints.ALFA  BreakpointsForDimension2=admireDB.aerodata_asym_ext.CRMRAL.breakpoints.DN  BreakpointsForDimension3=[5, 7]  Table=admireDB.aerodata_asym_ext.CRMRAL.newTable  ExtrapMethod=Clip  InternalRulePriority=Speed  RndMeth=Simplest  InputSameDT=on
      settings: InputPortMap=u0,u1
  Product : Product  Inputs=**
  Crmr : Outport
  wires:
  CRMRAL_DN_ALFA/1 -> Product/1
  angleOfAttack_deg/1 -> CRMRAL_DN_ALFA/1
  dN/1 -> CRMRAL_DN_ALFA/2
  Product/1 -> Crmr/1
  rc/1 -> Product/2

== system kamerol/Aerodynamics/RollMomentCoefficient/MachRegion1/Crmrbeta/Crmrbeta_ ==
  angleOfSideslip_deg : Inport
  angleOfAttack_deg : Inport  Port=2
  rc : Inport  Port=3
  Abs : Abs
  CRMRBA_BETA_ALFA : Lookup_n-D  BreakpointsForDimension1=admireDB.aerodata_asym_ext.CRMRBA.breakpoints.ALFA  BreakpointsForDimension2=admireDB.aerodata_asym_ext.CRMRBA.breakpoints.BETA  BreakpointsForDimension3=[5, 7]  Table=admireDB.aerodata_asym_ext.CRMRBA.newTable  ExtrapMethod=Clip  InternalRulePriority=Speed  RndMeth=Simplest  InputSameDT=on
      settings: InputPortMap=u0,u1
  Product : Product  Inputs=**
  Crmrbeta : Outport
  wires:
  Abs/1 -> CRMRBA_BETA_ALFA/2
  angleOfSideslip_deg/1 -> Abs/1
  angleOfAttack_deg/1 -> CRMRBA_BETA_ALFA/1
  rc/1 -> Product/2
  Product/1 -> Crmrbeta/1
  CRMRBA_BETA_ALFA/1 -> Product/1

== system kamerol/Aerodynamics/RollMomentCoefficient/MachRegion1/Crmrde/Crmrde_ ==
  mach_nd : Inport
  angleOfAttack_deg : Inport  Port=2
  rc : Inport  Port=3
  dEI : Inport  Port=4
  eieff : Inport  Port=5
  dey : Inport  Port=6
  eoeff : Inport  Port=7
  CRMRDEM_M : Lookup_n-D  NumberOfTableDimensions=1  BreakpointsForDimension1=admireDB.aerodata_asym_ext.CRMRDEM.breakpoints.M  BreakpointsForDimension3=[5, 7]  Table=admireDB.aerodata_asym_ext.CRMRDEM.newTable  ExtrapMethod=Clip  InternalRulePriority=Speed  RndMeth=Simplest  InputSameDT=on
  CRMRKA_ALFA : Lookup_n-D  NumberOfTableDimensions=1  BreakpointsForDimension1=admireDB.aerodata_asym_ext.CRMRKA.breakpoints.ALFA  BreakpointsForDimension3=[5, 7]  Table=admireDB.aerodata_asym_ext.CRMRKA.newTable  ExtrapMethod=Clip  InternalRulePriority=Speed  RndMeth=Simplest  InputSameDT=on
  Constant : Constant  Value=1/30
  Constant1 : Constant  Value=1/30
  Product : Product  Inputs=****
  Product1 : Product  Inputs=3
  Product2 : Product  Inputs=3
  Sum : Sum  Inputs=|++
  Crmrbeta : Outport
  wires:
  Sum/1 -> Product/4
  Product2/1 -> Sum/2
  Product1/1 -> Sum/1
  dey/1 -> Product2/1
  eoeff/1 -> Product2/3
  Constant1/1 -> Product2/2
  Constant/1 -> Product1/2
  eieff/1 -> Product1/3
  dEI/1 -> Product1/1
  CRMRKA_ALFA/1 -> Product/2
  CRMRDEM_M/1 -> Product/1
  mach_nd/1 -> CRMRDEM_M/1
  angleOfAttack_deg/1 -> CRMRKA_ALFA/1
  Product/1 -> Crmrbeta/1
  rc/1 -> Product/3

== system kamerol/Aerodynamics/RollMomentCoefficient/MachRegion2/Crmbasic/Crmbasic_ ==
  angleOfAttack_deg : Inport
  tflow : Inport  Port=2
  Abs : Abs
  CRMZERO_ALFA : Lookup_n-D  NumberOfTableDimensions=1  BreakpointsForDimension1=admireDB.aerodata_asym_ext.CRMZERO.breakpoints.ALFA  BreakpointsForDimension3=[5, 7]  Table=admireDB.aerodata_asym_ext.CRMZERO.newTable  ExtrapMethod=Clip  InternalRulePriority=Speed  RndMeth=Simplest  InputSameDT=on
  Product : Product
  Crmbasic : Outport
  wires:
  tflow/1 -> Product/2
  Product/1 -> Crmbasic/1
  CRMZERO_ALFA/1 -> Product/1
  angleOfAttack_deg/1 -> Abs/1
  Abs/1 -> CRMZERO_ALFA/1

== system kamerol/Aerodynamics/RollMomentCoefficient/MachRegion2/Crmbde/Crmbde_ ==
  angleOfAttack_deg : Inport
  dN : Inport  Port=2
  dEI : Inport  Port=3
  angleOfSideslip_deg : Inport  Port=4
  dEY : Inport  Port=5
  eieff : Inport  Port=6
  eoeff : Inport  Port=7
  Abs : Abs
  CRMDEB_ALFA_DN_DE_BETA : Lookup_n-D  NumberOfTableDimensions=4  BreakpointsForDimension1=admireDB.aerodata_asym_ext.CRMDEB.breakpoints.ALFA  BreakpointsForDimension2=admireDB.aerodata_asym_ext.CRMDEB.breakpoints.DN  BreakpointsForDimension3=admireDB.aerodata_asym_ext.CRMDEB.breakpoints.DE  BreakpointsForDimension4=admireDB.aerodata_asym_ext.CRMDEB.breakpoints.BETA  Table=admireDB.aerodata_asym_ext.CRMDEB.newTable  ExtrapMethod=Clip  InternalRulePriority=Speed  RndMeth=Simplest  InputSameDT=on
      settings: InputPortMap=u0,u1,u2,u3
  CRMDEB_ALFA_DN_DE_BETA1 : Lookup_n-D  NumberOfTableDimensions=4  BreakpointsForDimension1=admireDB.aerodata_asym_ext.CRMDEB.breakpoints.ALFA  BreakpointsForDimension2=admireDB.aerodata_asym_ext.CRMDEB.breakpoints.DN  BreakpointsForDimension3=admireDB.aerodata_asym_ext.CRMDEB.breakpoints.DE  BreakpointsForDimension4=admireDB.aerodata_asym_ext.CRMDEB.breakpoints.BETA  Table=admireDB.aerodata_asym_ext.CRMDEB.newTable  ExtrapMethod=Clip  InternalRulePriority=Speed  RndMeth=Simplest  InputSameDT=on
      settings: InputPortMap=u0,u1,u2,u3
  Product : Product  Inputs=**
  Product1 : Product  Inputs=**
  Product2 : Product
  Sign : Signum
  Sum : Sum  Inputs=|++
  Crmbde : Outport
  wires:
  dEY/1 -> CRMDEB_ALFA_DN_DE_BETA1/3
  dEI/1 -> CRMDEB_ALFA_DN_DE_BETA/3
  dN/1 -> CRMDEB_ALFA_DN_DE_BETA/2, CRMDEB_ALFA_DN_DE_BETA1/2
  angleOfAttack_deg/1 -> CRMDEB_ALFA_DN_DE_BETA/1, CRMDEB_ALFA_DN_DE_BETA1/1
  Abs/1 -> CRMDEB_ALFA_DN_DE_BETA1/4, CRMDEB_ALFA_DN_DE_BETA/4
  angleOfSideslip_deg/1 -> Sign/1, Abs/1
  CRMDEB_ALFA_DN_DE_BETA/1 -> Product/1
  CRMDEB_ALFA_DN_DE_BETA1/1 -> Product1/2
  eieff/1 -> Product/2
  eoeff/1 -> Product1/1
  Sum/1 -> Product2/2
  Product/1 -> Sum/1
  Product1/1 -> Sum/2
  Product2/1 -> Crmbde/1
  Sign/1 -> Product2/1

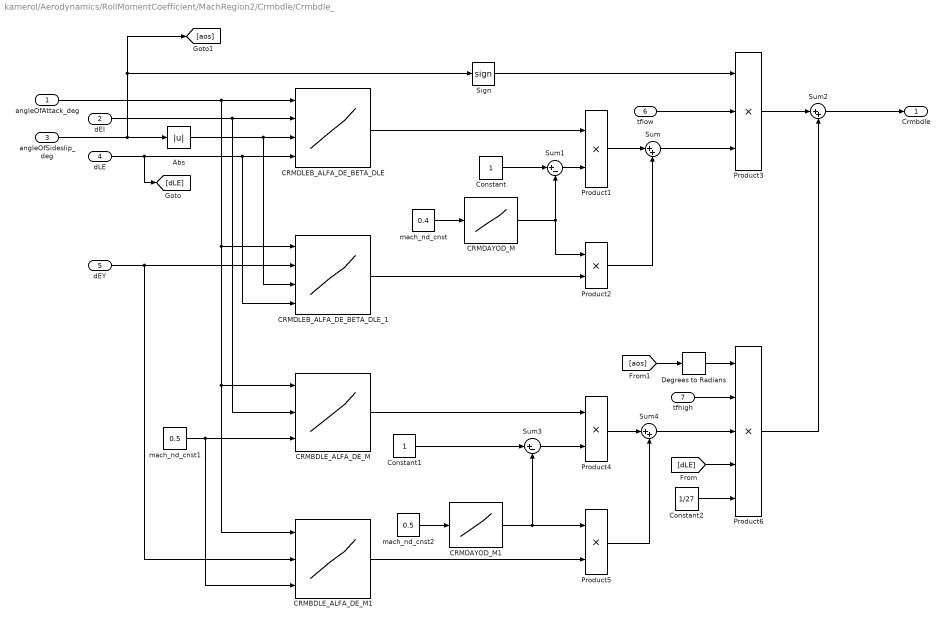
== system kamerol/Aerodynamics/RollMomentCoefficient/MachRegion2/Crmbdle/Crmbdle_ ==
  angleOfAttack_deg : Inport
  dEI : Inport  Port=2
  angleOfSideslip_deg : Inport  Port=3
  dLE : Inport  Port=4
  dEY : Inport  Port=5
  tflow : Inport  Port=6
  tfhigh : Inport  Port=7
  Abs : Abs
  CRMBDLE_ALFA_DE_M : Lookup_n-D  NumberOfTableDimensions=3  BreakpointsForDimension1=admireDB.aerodata_asym_ext.CRMBDLE.breakpoints.ALFA  BreakpointsForDimension2=admireDB.aerodata_asym_ext.CRMBDLE.breakpoints.DE  BreakpointsForDimension3=admireDB.aerodata_asym_ext.CRMBDLE.breakpoints.M  Table=admireDB.aerodata_asym_ext.CRMBDLE.newTable  ExtrapMethod=Clip  InternalRulePriority=Speed  RndMeth=Simplest  InputSameDT=on
      settings: InputPortMap=u0,u1,u2
  CRMBDLE_ALFA_DE_M1 : Lookup_n-D  NumberOfTableDimensions=3  BreakpointsForDimension1=admireDB.aerodata_asym_ext.CRMBDLE.breakpoints.ALFA  BreakpointsForDimension2=admireDB.aerodata_asym_ext.CRMBDLE.breakpoints.DE  BreakpointsForDimension3=admireDB.aerodata_asym_ext.CRMBDLE.breakpoints.M  Table=admireDB.aerodata_asym_ext.CRMBDLE.newTable  ExtrapMethod=Clip  InternalRulePriority=Speed  RndMeth=Simplest  InputSameDT=on
      settings: InputPortMap=u0,u1,u2
  CRMDAYOD_M : Lookup_n-D  NumberOfTableDimensions=1  BreakpointsForDimension1=admireDB.aerodata_asym_ext.CRMDAYOD.breakpoints.M  BreakpointsForDimension3=[5, 7]  Table=admireDB.aerodata_asym_ext.CRMDAYOD.newTable  ExtrapMethod=Clip  InternalRulePriority=Speed  RndMeth=Simplest  InputSameDT=on
  CRMDAYOD_M1 : Lookup_n-D  NumberOfTableDimensions=1  BreakpointsForDimension1=admireDB.aerodata_asym_ext.CRMDAYOD.breakpoints.M  BreakpointsForDimension3=[5, 7]  Table=admireDB.aerodata_asym_ext.CRMDAYOD.newTable  ExtrapMethod=Clip  InternalRulePriority=Speed  RndMeth=Simplest  InputSameDT=on
  CRMDLEB_ALFA_DE_BETA_DLE : Lookup_n-D  NumberOfTableDimensions=4  BreakpointsForDimension1=admireDB.aerodata_asym_ext.CRMDLEB.breakpoints.ALFA  BreakpointsForDimension2=admireDB.aerodata_asym_ext.CRMDLEB.breakpoints.DE  BreakpointsForDimension3=admireDB.aerodata_asym_ext.CRMDLEB.breakpoints.BETA  BreakpointsForDimension4=admireDB.aerodata_asym_ext.CRMDLEB.breakpoints.DLE  Table=admireDB.aerodata_asym_ext.CRMDLEB.newTable  ExtrapMethod=Clip  InternalRulePriority=Speed  RndMeth=Simplest  InputSameDT=on
      settings: InputPortMap=u0,u1,u2,u3
  CRMDLEB_ALFA_DE_BETA_DLE_1 : Lookup_n-D  NumberOfTableDimensions=4  BreakpointsForDimension1=admireDB.aerodata_asym_ext.CRMDLEB.breakpoints.ALFA  BreakpointsForDimension2=admireDB.aerodata_asym_ext.CRMDLEB.breakpoints.DE  BreakpointsForDimension3=admireDB.aerodata_asym_ext.CRMDLEB.breakpoints.BETA  BreakpointsForDimension4=admireDB.aerodata_asym_ext.CRMDLEB.breakpoints.DLE  Table=admireDB.aerodata_asym_ext.CRMDLEB.newTable  ExtrapMethod=Clip  InternalRulePriority=Speed  RndMeth=Simplest  InputSameDT=on
      settings: InputPortMap=u0,u1,u2,u3
  Constant : Constant
  Constant1 : Constant
  Constant2 : Constant  Value=1/27
  Degrees to Radians : simulink_extras/Transformations/Degrees to Radians
  Product1 : Product
  Product2 : Product  Inputs=**
  Product3 : Product  Inputs=3
  Product4 : Product  Inputs=**
  Product5 : Product  Inputs=**
  Product6 : Product  Inputs=5
  Sign : Signum
  Sum : Sum  Inputs=|++
  Sum1 : Sum  Inputs=|+-
  Sum2 : Sum  Inputs=|++
  Sum3 : Sum  Inputs=|+-
  Sum4 : Sum  Inputs=|++
  mach_nd_cnst : Constant  Value=0.4
  mach_nd_cnst1 : Constant  Value=0.5
  mach_nd_cnst2 : Constant  Value=0.5
  Crmbdle : Outport
  wires:
  mach_nd_cnst1/1 -> CRMBDLE_ALFA_DE_M1/3, CRMBDLE_ALFA_DE_M/3
  angleOfAttack_deg/1 -> CRMDLEB_ALFA_DE_BETA_DLE/1, CRMDLEB_ALFA_DE_BETA_DLE_1/1, CRMBDLE_ALFA_DE_M1/1, CRMBDLE_ALFA_DE_M/1
  Sum2/1 -> Crmbdle/1
  Product6/1 -> Sum2/2
  Constant2/1 -> Product6/5
  Degrees to Radians/1 -> Product6/1
  tfhigh/1 -> Product6/2
  [dLE] -> Product6/4
  [aos] -> Degrees to Radians/1
  Sum4/1 -> Product6/3
  Product5/1 -> Sum4/2
  CRMBDLE_ALFA_DE_M1/1 -> Product5/2
  Product4/1 -> Sum4/1
  Sum3/1 -> Product4/2
  CRMBDLE_ALFA_DE_M/1 -> Product4/1
  Constant1/1 -> Sum3/1
  CRMDAYOD_M1/1 -> Product5/1, Sum3/2
  mach_nd_cnst2/1 -> CRMDAYOD_M1/1
  dEI/1 -> CRMDLEB_ALFA_DE_BETA_DLE/2, CRMBDLE_ALFA_DE_M/2
  tflow/1 -> Product3/2
  Sum/1 -> Product3/3
  Product2/1 -> Sum/2
  Product1/1 -> Sum/1
  Sum1/1 -> Product1/2
  mach_nd_cnst/1 -> CRMDAYOD_M/1
  CRMDAYOD_M/1 -> Sum1/2, Product2/1
  Constant/1 -> Sum1/1
  Product3/1 -> Sum2/1
  dEY/1 -> CRMBDLE_ALFA_DE_M1/2, CRMDLEB_ALFA_DE_BETA_DLE_1/2
  angleOfSideslip_deg/1 -> [aos], Sign/1, Abs/1
  dLE/1 -> CRMDLEB_ALFA_DE_BETA_DLE_1/4, CRMDLEB_ALFA_DE_BETA_DLE/4, [dLE]
  Abs/1 -> CRMDLEB_ALFA_DE_BETA_DLE_1/3, CRMDLEB_ALFA_DE_BETA_DLE/3
  Sign/1 -> Product3/1
  CRMDLEB_ALFA_DE_BETA_DLE_1/1 -> Product2/2
  CRMDLEB_ALFA_DE_BETA_DLE/1 -> Product1/1

== system kamerol/Aerodynamics/RollMomentCoefficient/MachRegion2/Crmbdn/Crmbdn_ ==
  angleOfSideslip_deg : Inport
  dN : Inport  Port=2
  angleOfAttack_deg : Inport  Port=3
  tflow : Inport  Port=4
  tfhigh : Inport  Port=5
  Abs : Abs
  CRMBMDN_DN_M : Lookup_n-D  BreakpointsForDimension1=admireDB.aerodata_asym_ext.CRMBMDN.breakpoints.M  BreakpointsForDimension2=admireDB.aerodata_asym_ext.CRMBMDN.breakpoints.DN  BreakpointsForDimension3=[5, 7]  Table=admireDB.aerodata_asym_ext.CRMBMDN.newTable  ExtrapMethod=Clip  InternalRulePriority=Speed  RndMeth=Simplest  InputSameDT=on
      settings: InputPortMap=u0,u1
  CRMDNB_ALFA_DN_BETA : Lookup_n-D  NumberOfTableDimensions=3  BreakpointsForDimension1=admireDB.aerodata_asym_ext.CRMDNB.breakpoints.ALFA  BreakpointsForDimension2=admireDB.aerodata_asym_ext.CRMDNB.breakpoints.DN  BreakpointsForDimension3=admireDB.aerodata_asym_ext.CRMDNB.breakpoints.BETA  Table=admireDB.aerodata_asym_ext.CRMDNB.newTable  ExtrapMethod=Clip  InternalRulePriority=Speed  RndMeth=Simplest  InputSameDT=on
      settings: InputPortMap=u0,u1,u2
  Degrees to Radians : simulink_extras/Transformations/Degrees to Radians
  Product : Product  Inputs=3
  Product1 : Product  Inputs=***
  Sign : Signum
  Sum : Sum  Inputs=|++
  mach_nd_cnst : Constant  Value=0.5
  Crmbdn : Outport
  wires:
  angleOfAttack_deg/1 -> CRMDNB_ALFA_DN_BETA/1
  Abs/1 -> CRMDNB_ALFA_DN_BETA/3
  Sum/1 -> Crmbdn/1
  Product1/1 -> Sum/2
  tfhigh/1 -> Product1/2
  Degrees to Radians/1 -> Product1/3
  CRMBMDN_DN_M/1 -> Product1/1
  mach_nd_cnst/1 -> CRMBMDN_DN_M/1
  angleOfSideslip_deg/1 -> Sign/1, Degrees to Radians/1, Abs/1
  dN/1 -> CRMBMDN_DN_M/2, CRMDNB_ALFA_DN_BETA/2
  tflow/1 -> Product/2
  Product/1 -> Sum/1
  CRMDNB_ALFA_DN_BETA/1 -> Product/3
  Sign/1 -> Product/1

== system kamerol/Aerodynamics/RollMomentCoefficient/MachRegion2/Crmbeta/Crmbeta_ ==
  angleOfSideslip_deg : Inport
  angleOfAttack_deg : Inport  Port=2
  tflow : Inport  Port=3
  thigh : Inport  Port=4
  qacorr : Inport  Port=5
  mach_nd : Inport  Port=6
  Abs : Abs
  CRMBAL_BETA_ALFA : Lookup_n-D  BreakpointsForDimension1=admireDB.aerodata_asym_ext.CRMBAL.breakpoints.ALFA  BreakpointsForDimension2=admireDB.aerodata_asym_ext.CRMBAL.breakpoints.BETA  BreakpointsForDimension3=[5, 7]  Table=admireDB.aerodata_asym_ext.CRMBAL.newTable  ExtrapMethod=Clip  InternalRulePriority=Speed  RndMeth=Simplest  InputSameDT=on
      settings: InputPortMap=u0,u1
  CRMBMA_M_ALFA : Lookup_n-D  BreakpointsForDimension1=admireDB.aerodata_asym_ext.CRMBMA.breakpoints.ALFA  BreakpointsForDimension2=admireDB.aerodata_asym_ext.CRMBMA.breakpoints.M  BreakpointsForDimension3=[5, 7]  Table=admireDB.aerodata_asym_ext.CRMBMA.newTable  ExtrapMethod=Clip  InternalRulePriority=Speed  RndMeth=Simplest  InputSameDT=on
      settings: InputPortMap=u0,u1
  CRMEB_QA_M : Lookup_n-D  BreakpointsForDimension1=admireDB.aerodata_asym_ext.CRMEB.breakpoints.M  BreakpointsForDimension2=admireDB.aerodata_asym_ext.CRMEB.breakpoints.QA  BreakpointsForDimension3=[5, 7]  Table=admireDB.aerodata_asym_ext.CRMEB.newTable  ExtrapMethod=Clip  InternalRulePriority=Speed  RndMeth=Simplest  InputSameDT=on
      settings: InputPortMap=u0,u1
  Degrees to Radians : simulink_extras/Transformations/Degrees to Radians
  Product : Product  Inputs=3
  Product1 : Product
  Product2 : Product  Inputs=3
  Sign : Signum
  Sum : Sum  Inputs=+++
  mach_nd_cnst : Constant  Value=0.5
  Crmbeta : Outport
  wires:
  Product2/1 -> Sum/2
  thigh/1 -> Product2/1
  CRMBMA_M_ALFA/1 -> Product2/2
  mach_nd_cnst/1 -> CRMBMA_M_ALFA/2
  angleOfAttack_deg/1 -> CRMBAL_BETA_ALFA/1, CRMBMA_M_ALFA/1
  tflow/1 -> Product/3
  qacorr/1 -> CRMEB_QA_M/2
  mach_nd/1 -> CRMEB_QA_M/1
  angleOfSideslip_deg/1 -> Abs/1, Sign/1, Degrees to Radians/1
  CRMBAL_BETA_ALFA/1 -> Product/2
  Sign/1 -> Product/1
  Abs/1 -> CRMBAL_BETA_ALFA/2
  Product/1 -> Sum/1
  CRMEB_QA_M/1 -> Product1/2
  Degrees to Radians/1 -> Product1/1, Product2/3
  Product1/1 -> Sum/3
  Sum/1 -> Crmbeta/1

== system kamerol/Aerodynamics/RollMomentCoefficient/MachRegion2/Crmbetad/Crmbetad_ ==
  angleOfAttack_deg : Inport
  betad : Inport  Port=2
  tflow : Inport  Port=3
  tfhigh : Inport  Port=4
  CRMBDH_ALFA_M : Lookup_n-D  BreakpointsForDimension1=admireDB.aerodata_asym_ext.CRMBDH.breakpoints.M  BreakpointsForDimension2=admireDB.aerodata_asym_ext.CRMBDH.breakpoints.ALFA  BreakpointsForDimension3=[5, 7]  Table=admireDB.aerodata_asym_ext.CRMBDH.newTable  ExtrapMethod=Clip  InternalRulePriority=Speed  RndMeth=Simplest  InputSameDT=on
      settings: InputPortMap=u0,u1
  CRMBDL_ALFA : Lookup_n-D  NumberOfTableDimensions=1  BreakpointsForDimension1=admireDB.aerodata_asym_ext.CRMBDL.breakpoints.ALFA  BreakpointsForDimension3=[5, 7]  Table=admireDB.aerodata_asym_ext.CRMBDL.newTable  ExtrapMethod=Clip  InternalRulePriority=Speed  RndMeth=Simplest  InputSameDT=on
  Product : Product  Inputs=**
  Product1 : Product  Inputs=**
  Product2 : Product  Inputs=**
  Sum : Sum  Inputs=|++
  mach_nd_cnst : Constant  Value=0.5
  Crmbetad : Outport
  wires:
  Sum/1 -> Product/1
  Product1/1 -> Sum/1
  Product2/1 -> Sum/2
  tfhigh/1 -> Product2/1
  tflow/1 -> Product1/2
  CRMBDH_ALFA_M/1 -> Product2/2
  mach_nd_cnst/1 -> CRMBDH_ALFA_M/1
  betad/1 -> Product/2
  CRMBDL_ALFA/1 -> Product1/1
  Product/1 -> Crmbetad/1
  angleOfAttack_deg/1 -> CRMBDL_ALFA/1, CRMBDH_ALFA_M/2

== system kamerol/Aerodynamics/RollMomentCoefficient/MachRegion2/Crmblg/Crmblg_ ==
  dLG : Inport
  angleOfAttack_deg : Inport  Port=2
  angleOfSideslip_deg : Inport  Port=3
  CRMBLST_NG_DOOR_ALFA : Lookup_n-D  BreakpointsForDimension1=admireDB.aerodata_asym_ext.CRMBLST.breakpoints.ALFA  BreakpointsForDimension2=admireDB.aerodata_asym_ext.CRMBLST.breakpoints.NG_DOOR  BreakpointsForDimension3=[5, 7]  Table=admireDB.aerodata_asym_ext.CRMBLST.newTable  ExtrapMethod=Clip  InternalRulePriority=Speed  RndMeth=Simplest  InputSameDT=on
      settings: InputPortMap=u0,u1
  Degrees to Radians : simulink_extras/Transformations/Degrees to Radians
  Product : Product  Inputs=3
  Crmblg : Outport
  wires:
  angleOfSideslip_deg/1 -> Degrees to Radians/1
  Product/1 -> Crmblg/1
  angleOfAttack_deg/1 -> CRMBLST_NG_DOOR_ALFA/1
  dLG/1 -> CRMBLST_NG_DOOR_ALFA/2, Product/1
  CRMBLST_NG_DOOR_ALFA/1 -> Product/2
  Degrees to Radians/1 -> Product/3
